simulink model "monopod_leg_force"  (R2013a)
settings: Solver=FixedStepDiscrete  StartTime=0.0  StopTime=inf  FixedStep=sample_time  RelTol=1e-3
InitFcn:
  | init_monopod_leg_force;
values from neighbouring files (symbols this model uses):
  sample_time = 1/update_freq    (= 0.001)    [init_monopod_leg_force.m]
undefined symbols (not defined in the file or in its folder): BOOM_MAX_ENCODER_TICKS, boom_mount_angle, BOOM_PITCH_CAL_VALUE_RAD, BOOM_PITCH_CAL_VALUE_TICKS, BOOM_PITCH_ENCODER_RAD_PER_TICK, BOOM_ROLL_CAL_VALUE_RAD, BOOM_ROLL_CAL_VALUE_TICKS, BOOM_ROLL_ENCODER_RAD_PER_TICK, BOOM_YAW_ENCODER_RAD_PER_TICK, control_start_time, DiscIntNeverNeededParam, fcut_acceleration, fcut_smooth, fcut_unwrap, fcut_velocity, HIP_ABS_ENCODER_RAD_PER_TICK, HIP_ABS_MAX_ENCODER_TICKS, hip_gravity_compensation, HIP_INC_ENCODER_RAD_PER_TICK, HIP_INC_MAX_ENCODER_TICKS, HIP_MOTOR_CONSTANT, HIP_MTR_GEAR_RATIO, HIP_MTR_MAX_TORQUE, i_limit_lateral, j_rotor_reflected, k_ff, k_sea, k_virtual, kd_lateral, kd_leg_angle, kd_sea_torque, ki_lateral, kp_lateral, kp_leg_angle, kp_sea_torque, l0_virtual, l_seg, lateral_torque_ramp_time, LEFT_HIP_CALIB_POS, LEFT_HIP_CALIB_VAL, LEFT_MOTOR_HIP_DIRECTION, LEG1_LEG_A_CALIB_VAL, LEG1_LEG_A_RAD_PER_CNT, LEG1_LEG_B_CALIB_VAL, LEG1_LEG_B_RAD_PER_CNT, LEG1_MOTOR_A_DIRECTION, LEG1_MOTOR_B_DIRECTION, LEG1_TRAN_A_CALIB_VAL, LEG1_TRAN_A_RAD_PER_CNT, LEG1_TRAN_B_CALIB_VAL, LEG1_TRAN_B_RAD_PER_CNT, LEG2_LEG_A_CALIB_VAL, LEG2_LEG_A_RAD_PER_CNT, LEG2_LEG_B_CALIB_VAL, LEG2_LEG_B_RAD_PER_CNT, LEG2_MOTOR_A_DIRECTION, LEG2_MOTOR_B_DIRECTION, LEG2_TRAN_A_CALIB_VAL, LEG2_TRAN_A_RAD_PER_CNT, LEG2_TRAN_B_CALIB_VAL ... (+18)
libraries: xpcethercatlib x160, simulink x13, dspswit3 x1
(part 3 of 3)

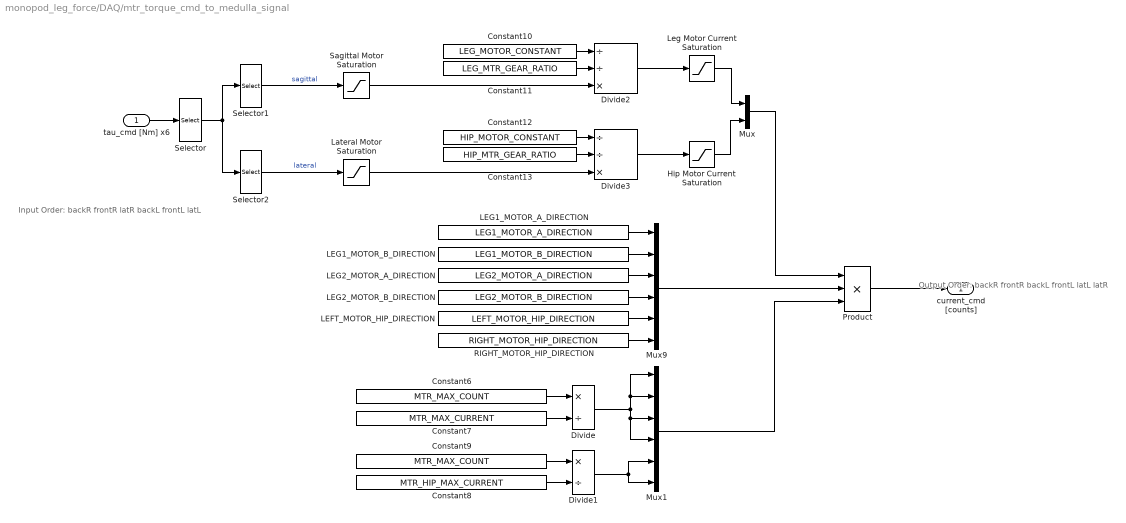
== system monopod_leg_force/DAQ/mtr_torque_cmd_to_medulla_signal ==
  note: Output Order:
      |
      | backR
      | frontR
      | backL
      | frontL
      | latL
      | latR
  note: Input Order:
      |
      | backR
      | frontR
      | latR
      | backL
      | frontL
      | latL
  tau_cmd [Nm] x6 : Inport
  Constant10 : Constant  Value=LEG_MOTOR_CONSTANT
  Constant11 : Constant  Value=LEG_MTR_GEAR_RATIO
  Constant12 : Constant  Value=HIP_MOTOR_CONSTANT
  Constant13 : Constant  Value=HIP_MTR_GEAR_RATIO
  Constant6 : Constant  Value=MTR_MAX_COUNT
  Constant7 : Constant  Value=MTR_MAX_CURRENT
  Constant8 : Constant  Value=MTR_HIP_MAX_CURRENT
  Constant9 : Constant  Value=MTR_MAX_COUNT
  Divide : Product  Inputs=*/
  Divide1 : Product  Inputs=*/
  Divide2 : Product  Inputs=//*
  Divide3 : Product  Inputs=//*
  Hip Motor Current Saturation : Saturate  UpperLimit=10  LowerLimit=-10
      settings: AttributesFormatString=Top: %<UpperLimit>\nBottom: %<LowerLimit>
  LEFT_MOTOR_HIP_DIRECTION : Constant  Value=LEFT_MOTOR_HIP_DIRECTION
  LEG1_MOTOR_A_DIRECTION : Constant  Value=LEG1_MOTOR_A_DIRECTION
  LEG1_MOTOR_B_DIRECTION : Constant  Value=LEG1_MOTOR_B_DIRECTION
  LEG2_MOTOR_A_DIRECTION : Constant  Value=LEG2_MOTOR_A_DIRECTION
  LEG2_MOTOR_B_DIRECTION : Constant  Value=LEG2_MOTOR_B_DIRECTION
  Lateral Motor Saturation : Saturate  UpperLimit=HIP_MTR_MAX_TORQUE  LowerLimit=-HIP_MTR_MAX_TORQUE
      settings: AttributesFormatString=Top: %<UpperLimit>\nBottom: %<LowerLimit>
  Leg Motor Current Saturation : Saturate  UpperLimit=30  LowerLimit=-30
      settings: AttributesFormatString=Top: %<UpperLimit>\nBottom: %<LowerLimit>
  Mux : Mux  Inputs=2
  Mux1 : Mux  Inputs=6
  Mux9 : Mux  Inputs=6
  Product : Product  Inputs=3  RndMeth=Zero
  RIGHT_MOTOR_HIP_DIRECTION : Constant  Value=RIGHT_MOTOR_HIP_DIRECTION
  Sagittal Motor Saturation : Saturate  UpperLimit=LEG_MTR_MAX_TORQUE  LowerLimit=-LEG_MTR_MAX_TORQUE
      settings: AttributesFormatString=Top: %<UpperLimit>\nBottom: %<LowerLimit>
  Selector : Selector  InputPortWidth=6  IndexOptions=Index vector (dialog)  Indices=[1 2 4 5 6 3]  OutputSizes=1
  Selector1 : Selector  InputPortWidth=6  IndexOptions=Index vector (dialog)  Indices=[1 2 3 4]  OutputSizes=1
  Selector2 : Selector  InputPortWidth=6  IndexOptions=Index vector (dialog)  Indices=[5 6]  OutputSizes=1
  current_cmd [counts] : Outport
  wires:
  Lateral Motor Saturation/1 -> Divide3/3
  Sagittal Motor Saturation/1 -> Divide2/3
  Hip Motor Current Saturation/1 -> Mux/2
  Leg Motor Current Saturation/1 -> Mux/1
  Mux/1 -> Product/1
  Divide2/1 -> Leg Motor Current Saturation/1
  Divide3/1 -> Hip Motor Current Saturation/1
  Constant12/1 -> Divide3/1
  Constant13/1 -> Divide3/2
  Constant10/1 -> Divide2/1
  Constant11/1 -> Divide2/2
  Selector2/1 -> Lateral Motor Saturation/1  "lateral"
  Selector1/1 -> Sagittal Motor Saturation/1  "sagittal"
  LEG1_MOTOR_A_DIRECTION/1 -> Mux9/1
  LEG1_MOTOR_B_DIRECTION/1 -> Mux9/2
  LEG2_MOTOR_A_DIRECTION/1 -> Mux9/3
  Mux9/1 -> Product/2
  LEG2_MOTOR_B_DIRECTION/1 -> Mux9/4
  LEFT_MOTOR_HIP_DIRECTION/1 -> Mux9/5
  RIGHT_MOTOR_HIP_DIRECTION/1 -> Mux9/6
  Product/1 -> current_cmd [counts]/1
  Constant6/1 -> Divide/1
  Constant7/1 -> Divide/2
  Divide/1 -> Mux1/4, Mux1/3, Mux1/2, Mux1/1
  Constant9/1 -> Divide1/1
  Constant8/1 -> Divide1/2
  Divide1/1 -> Mux1/6, Mux1/5
  Mux1/1 -> Product/3
  tau_cmd [Nm] x6/1 -> Selector/1
  Selector/1 -> Selector1/1, Selector2/1

== system monopod_leg_force/DAQ/remove_encoder_dropouts ==
  note: Predict Behavior of Signal
  note: predicted value:
      | phi' = phi_(n-1) + dphi
      | = phi_(n-1) + phi_(n-1)-phi_(n-2)
  measured : Inport
  Abs : Abs
  Clock : Clock
  Compare To Zero1 : simulink/Logic and Bit Operations/Compare To Zero  relop=>  OutDataTypeStr=boolean
  Constant : Constant  Value=sensor_start_time+2*sample_time
  Discrete Single Pole Lowpass Filter : DiscreteTransferFcn  Numerator=[(1-exp(-2*pi*fcut_smooth*sample_time)) 0]  Denominator=[1 -exp(-2*pi*fcut_smooth*sample_time)]  SampleTime=sample_time
  Gain2 : Gain  Gain=2
  Sum : Sum  Inputs=|+-
  Sum2 : Sum  Inputs=|+-
  Sum3 : Sum  Inputs=-+|
  Switch : Switch  Criteria=u2 ~= 0  Threshold=max_sensor_velocity*sample_time
      settings: AttributesFormatString=%<Criteria>
  Unit Delay phi_(n-1) : UnitDelay  SampleTime=-1
      settings: AttributesFormatString=initial condition = %<X0>
  Unit Delay phi_(n-2) : UnitDelay  SampleTime=-1
      settings: AttributesFormatString=initial condition = %<X0>
  check_error : Subsystem
  smoothed : Outport
  wires:
  Compare To Zero1/1 -> check_error/Enable
  Constant/1 -> Sum2/2
  Clock/1 -> Sum2/1
  Sum2/1 -> Compare To Zero1/1
  check_error/1(acceptable?) -> Switch/2
  Sum3/1 -> Abs/1  "error"
  Abs/1 -> check_error/1(error)
  Discrete Single Pole Lowpass Filter/1 -> Unit Delay phi_(n-1)/1
  Switch/1 -> smoothed/1, Discrete Single Pole Lowpass Filter/1
  Unit Delay phi_(n-2)/1 -> Sum/2
  measured/1 -> Switch/1, Sum3/1  "phi"
  Unit Delay phi_(n-1)/1 -> Unit Delay phi_(n-2)/1, Gain2/1
  Gain2/1 -> Sum/1
  Sum/1 -> Sum3/2, Switch/3  "phi'"

== system monopod_leg_force/DAQ/unwrap_encoders ==
  Encoder Readings : Inport
  Demux : Demux  Outputs=5
  Mux : Mux  Inputs=6
  Selector : Selector  InputPortWidth=15  IndexOptions=Index vector (dialog)  Indices=[9 10 11 12 14]  OutputSizes=1
  Selector1 : Selector  InputPortWidth=20  IndexOptions=Index vector (dialog)  Indices=[1 2 3 4 5 6 7 8 16 17 18 19 13 20 15]  OutputSizes=1
  unwrap_boom_yaw_encoder : Subsystem
  unwrap_lateral_absolute_encoders Left : Subsystem
  unwrap_lateral_absolute_encoders Right : Subsystem
  unwrap_lateral_incremental_encoders Left : Subsystem
  unwrap_lateral_incremental_encoders Right : Subsystem
  Adjusted Encoder Readings : Outport
  wires:
  Encoder Readings/1 -> Mux/1, Selector/1
  Selector/1 -> Demux/1
  Demux/2 -> unwrap_lateral_incremental_encoders Left/1(wrapped [ticks])
  Demux/4 -> unwrap_lateral_incremental_encoders Right/1(wrapped [ticks])
  Demux/5 -> unwrap_boom_yaw_encoder/1(wrapped [ticks])
  unwrap_lateral_incremental_encoders Left/1(continuous [ticks]) -> Mux/3
  unwrap_lateral_incremental_encoders Right/1(continuous [ticks]) -> Mux/5
  unwrap_boom_yaw_encoder/1(continuous [ticks]) -> Mux/6
  Selector1/1 -> Adjusted Encoder Readings/1
  Mux/1 -> Selector1/1
  Demux/1 -> unwrap_lateral_absolute_encoders Left/1(wrapped [ticks])
  Demux/3 -> unwrap_lateral_absolute_encoders Right/1(wrapped [ticks])
  unwrap_lateral_absolute_encoders Right/1(continuous [ticks]) -> Mux/4
  unwrap_lateral_absolute_encoders Left/1(continuous [ticks]) -> Mux/2

== system monopod_leg_force/Control/Actuator Control/SEA Controller ==
  phi_load [rad] x4 : Inport
  phi_gear [rad] x4 : Inport  Port=2
  tau_des sagittal [Nm] x4 : Inport  Port=3
  dphi_load [rad/s] x4 : Inport  Port=4
  dphi_gear [rad/s] x4 : Inport  Port=5
  Constant : Constant  Value=0
  Constant1 : Constant  Value=0
  Constant3 : Constant
  Product : Product  SampleTime=sample_time  RndMeth=Zero
  Product1 : Product  RndMeth=Zero
  Spring Stiffness : Gain  Gain=k_sea
  Spring Stiffness1 : Gain  Gain=k_sea
  Sum : Sum  Inputs=|++  SampleTime=sample_time
  Sum1 : Sum  Inputs=-+|
  Sum2 : Sum  Inputs=|+-
  Sum3 : Sum  Inputs=+++
  Sum5 : Sum  Inputs=|+-
  Sum6 : Sum  Inputs=-+|
  Sum7 : Sum  Inputs=|++
  Torque Limiter (outside) 1 : Saturate  UpperLimit=max_sagittal_torque  LowerLimit=-max_sagittal_torque
      settings: AttributesFormatString=Hi: %<UpperLimit>\nLo: %<LowerLimit>
  filtered_derivative : Subsystem
  j_motor : Gain  Description=xPCTag(1)=kd_sea_torque;  Gain=j_rotor_reflected
  k_ff : Gain  Gain=k_ff
  kd_gain : Gain  Description=xPCTag(1)=kd_sea_torque;  Gain=kd_sea_torque
  kp_gain : Constant  Description=xPCTag(1)=kp_sea_torque;  Value=kp_sea_torque  SampleTime=sample_time
  tau_cmd sagittal [Nm] x4 : Outport
  wires:
  Torque Limiter (outside) 1/1 -> tau_cmd sagittal [Nm] x4/1
  j_motor/1 -> k_ff/1
  filtered_derivative/1(dx/dt) -> j_motor/1
  Sum/1 -> Product1/2
  Constant3/1 -> Sum/2
  Sum7/1 -> Sum3/2
  kd_gain/1 -> Sum7/2
  Product/1 -> Sum7/1
  Sum5/1 -> Product/2
  Sum2/1 -> kd_gain/1
  dphi_gear [rad/s] x4/1 -> Sum6/2
  dphi_load [rad/s] x4/1 -> filtered_derivative/1(x), Sum6/1
  Spring Stiffness1/1 -> Sum2/2
  Sum6/1 -> Spring Stiffness1/1
  Constant1/1 -> Sum2/1
  Constant/1 -> Sum5/1
  phi_gear [rad] x4/1 -> Sum1/2
  phi_load [rad] x4/1 -> Sum1/1
  Sum3/1 -> Torque Limiter (outside) 1/1
  Product1/1 -> Sum3/1
  tau_des sagittal [Nm] x4/1 -> Product1/1
  Spring Stiffness/1 -> Sum5/2
  Sum1/1 -> Spring Stiffness/1
  kp_gain/1 -> Sum/1, Product/1
  k_ff/1 -> Sum3/3

== system monopod_leg_force/Control/Actuator Control/ramped_signal ==
  cmd : Inport
  Constant : Constant  Value=0
  Demux : Demux
  Mux1 : Mux
  Mux6 : Mux  Inputs=2
  Product : Product  RndMeth=Zero
  Product1 : Product  RndMeth=Zero
  Ramp : simulink/Sources/Ramp  slope=1/sagittal_torque_ramp_time  start=sagittal_starting_time  X0=0
      settings: AttributesFormatString=Start: %<start>\nSlope: %<slope>
  Ramp1 : simulink/Sources/Ramp  slope=1/lateral_torque_ramp_time  start=control_start_time  X0=0
      settings: AttributesFormatString=Start: %<start>\nSlope: %<slope>
  Saturation : Saturate  UpperLimit=1  LowerLimit=0
      settings: AttributesFormatString=Hi: %<UpperLimit>\nLo: %<LowerLimit>
  Saturation1 : Saturate  UpperLimit=1  LowerLimit=0
      settings: AttributesFormatString=Hi: %<UpperLimit>\nLo: %<LowerLimit>
  Selector10 : Selector  InputPortWidth=6  IndexOptions=Index vector (dialog)  Indices=[1 2 4 5]  OutputSizes=1
  Selector34 : Selector  InputPortWidth=6  IndexOptions=Index vector (dialog)  Indices=[1 2 5 3 4 6]  OutputSizes=1
  Selector9 : Selector  InputPortWidth=6  IndexOptions=Index vector (dialog)  Indices=[3 6]  OutputSizes=1
  Terminator : Terminator
  Terminator1 : Terminator
  ramped_cmd : Outport
  wires:
  Demux/3 -> Terminator1/1
  Demux/4 -> Terminator/1
  Constant/1 -> Mux1/4, Mux1/3
  Mux1/1 -> Product/1
  Demux/2 -> Mux1/2
  Demux/1 -> Mux1/1
  Mux6/1 -> Selector34/1
  Selector10/1 -> Demux/1
  Selector34/1 -> ramped_cmd/1
  Product1/1 -> Mux6/2
  cmd/1 -> Selector9/1, Selector10/1
  Product/1 -> Mux6/1
  Ramp/1 -> Saturation/1
  Saturation/1 -> Product/2
  Ramp1/1 -> Saturation1/1
  Saturation1/1 -> Product1/2
  Selector9/1 -> Product1/1

== system monopod_leg_force/Control/Behavior Control/Lateral PID Control ==
  q_cmu : Inport
  dq_cmu : Inport  Port=2
  Gain : Gain  Gain=-1
  Lateral Hip PID : Subsystem
  Motor Saturation : Saturate  UpperLimit=max_torque_lateral  LowerLimit=-max_torque_lateral
      settings: AttributesFormatString=Top: %<UpperLimit>\nBottom: %<LowerLimit>
  Mux : Mux  Inputs=2
  Sum1 : Sum  Inputs=|+-
  Sum2 : Sum  Inputs=|+-
  Sum4 : Sum  Inputs=++|
  desired_velocity : Constant  Value=0
  feedforward_torque (gravity compensation) : Constant  Value=hip_gravity_compensation
  select_dqLateral : Selector  InputPortWidth=13  IndexOptions=Index vector (dialog)  Indices=[9 10]  OutputSizes=1
  select_qLateral : Selector  InputPortWidth=13  IndexOptions=Index vector (dialog)  Indices=[9 10]  OutputSizes=1
  spherical_correction_angle : Subsystem
  tau_lateral : Outport
  wires:
  spherical_correction_angle/1(lateral_correction [rad]) -> Mux/1, Gain/1
  Lateral Hip PID/1(out) -> Sum4/2
  Sum2/1 -> Lateral Hip PID/1(position_error)
  q_cmu/1 -> spherical_correction_angle/1(q_cmu), select_qLateral/1
  select_dqLateral/1 -> Sum1/2
  dq_cmu/1 -> select_dqLateral/1
  Sum4/1 -> Motor Saturation/1
  desired_velocity/1 -> Sum1/1
  Sum1/1 -> Lateral Hip PID/2(velocity_error)
  feedforward_torque (gravity compensation)/1 -> Sum4/1
  Gain/1 -> Mux/2
  Mux/1 -> Sum2/1
  select_qLateral/1 -> Sum2/2  "qLateral"
  Motor Saturation/1 -> tau_lateral/1

== system monopod_leg_force/Control/Behavior Control/Leg Calculator ==
  Front [rad rad/s] : Inport
  Back [rad rad/s] : Inport  Port=2
  Demux1 : Demux  Outputs=2
  Gain1 : Gain  Gain=2*l_seg
  Gain2 : Gain  Gain=l_seg
  Gain3 : Gain  Gain=-1
  Gain4 : Gain  Gain=0.5
  Gain5 : Gain  Gain=0.5
  Gain6 : Gain  Gain=2
  Mux1 : Mux  Inputs=2
  Product : Product  RndMeth=Zero
  Sum4 : Sum  Inputs=+|+
  Sum5 : Sum  Inputs=+|-
  Trigonometric Function : Trigonometry  Operator=cos
  Trigonometric Function1 : Trigonometry
  "Leg Length [m m/s] " : Outport
  Leg Angle [rad rad/s] : Outport  Port=2
  Leg Splay [rad rad/s] : Outport  Port=3
  w [m] : Outport  Port=4
  wires:
  Gain6/1 -> w [m]/1
  Gain4/1 -> Trigonometric Function1/1, Trigonometric Function/1
  Trigonometric Function/1 -> Gain1/1
  Gain1/1 -> Mux1/1
  Trigonometric Function1/1 -> Gain2/1
  Product/1 -> Mux1/2
  Front [rad rad/s]/1 -> Sum5/2, Sum4/2
  Back [rad rad/s]/1 -> Sum4/1, Sum5/1
  Demux1/2 -> Gain3/1
  Gain3/1 -> Product/2
  Demux1/1 -> Gain4/1
  Gain2/1 -> Product/1, Gain6/1
  Sum5/1 -> Leg Splay [rad rad/s]/1, Demux1/1
  Mux1/1 -> "Leg Length [m m/s] "/1
  Sum4/1 -> Gain5/1
  Gain5/1 -> Leg Angle [rad rad/s]/1

== system monopod_leg_force/Control/Behavior Control/R Leg Angle PD ==
  Desired Angle : Inport
  Desired Velocity : Inport  Port=2
  Leg Angle [rad rad/s] : Inport  Port=3
  Demux1 : Demux  Outputs=2
  Gain6 : Gain  Gain=kp_leg_angle
  Gain7 : Gain  Gain=kd_leg_angle
  Sum7 : Sum  Inputs=|+-
  Sum8 : Sum  Inputs=|+-
  Sum9 : Sum  Inputs=|++
  Commanded Leg Torque [Nm] : Outport
  wires:
  Sum7/1 -> Gain6/1
  Demux1/1 -> Sum7/2
  Sum9/1 -> Commanded Leg Torque [Nm]/1
  Desired Velocity/1 -> Sum8/1
  Sum8/1 -> Gain7/1
  Desired Angle/1 -> Sum7/1
  Demux1/2 -> Sum8/2
  Leg Angle [rad rad/s]/1 -> Demux1/1
  Gain6/1 -> Sum9/1
  Gain7/1 -> Sum9/2

== system monopod_leg_force/Control/Behavior Control/Torque Distribution ==
  Leg Torque [Nm] : Inport
  Leg Force [N] : Inport  Port=2
  Leg Splay [rad] : Inport  Port=3
  Gain : Gain  Gain=0.5
  Gain1 : Gain  Gain=0.5
  Gain2 : Gain  Gain=2*l_seg
  Gain3 : Gain  Gain=0.5
  Product : Product  RndMeth=Zero
  Sum : Sum  Inputs=|++
  Sum1 : Sum  Inputs=+-|
  Trigonometric Function1 : Trigonometry
  Back Torque [Nm] : Outport
  Front Torque [Nm] : Outport  Port=2
  wires:
  Sum1/1 -> Back Torque [Nm]/1
  Leg Torque [Nm]/1 -> Gain/1
  Sum/1 -> Front Torque [Nm]/1
  Gain/1 -> Sum/1, Sum1/1
  Gain3/1 -> Trigonometric Function1/1
  Leg Splay [rad]/1 -> Gain3/1
  Trigonometric Function1/1 -> Gain2/1
  Gain2/1 -> Product/2  "w [m]"
  Gain1/1 -> Sum1/2, Sum/2
  Leg Force [N]/1 -> Product/1
  Product/1 -> Gain1/1

== system monopod_leg_force/DAQ/calibrate_and_convert_to_rad/calibrate_abs_encoder ==
  encoder_ticks : Inport
  cal_pt_ticks : Inport  Port=2
  cal_pt_rad : Inport  Port=3
  ticks_to_rad_const : Inport  Port=4
  Product : Product  RndMeth=Zero
  Sum : Sum  Inputs=|+-
  Sum1 : Sum  Inputs=|++
  angle [rad] : Outport
  wires:
  cal_pt_rad/1 -> Sum1/2  "calibration_point_radians"
  Sum1/1 -> angle [rad]/1  "calibrated_angle"
  cal_pt_ticks/1 -> Sum/2  "calibration_point_ticks"
  ticks_to_rad_const/1 -> Product/2  "ticks_to_rad_const"
  Product/1 -> Sum1/1  "rad_diff"
  encoder_ticks/1 -> Sum/1  "encoder_ticks"
  Sum/1 -> Product/1  "tick_diff"

== system monopod_leg_force/DAQ/calibrate_and_convert_to_rad/calibration_pt_radians ==
  Constant{1,3,5,7} (4 alike) : Constant  Value=LEG_A_CALIB_LOC
  Constant10 : Constant  Value=LEFT_HIP_CALIB_POS
  Constant11 : Constant  Value=BOOM_ROLL_CAL_VALUE_RAD
  Constant12 : Constant  Value=BOOM_PITCH_CAL_VALUE_RAD
  Constant{2,4,6,8} (4 alike) : Constant  Value=LEG_B_CALIB_LOC
  Constant9 : Constant  Value=RIGHT_HIP_CALIB_POS
  Mux3 : Mux  Inputs=12
  calibration_pt [rad] : Outport
  wires:
  Constant7/1 -> Mux3/5
  Constant10/1 -> Mux3/9
  Constant1/1 -> Mux3/2
  Constant5/1 -> Mux3/6
  Constant2/1 -> Mux3/3
  Constant9/1 -> Mux3/10
  Constant12/1 -> Mux3/12
  Constant6/1 -> Mux3/7
  Constant11/1 -> Mux3/11
  Mux3/1 -> calibration_pt [rad]/1
  Constant3/1 -> Mux3/1
  Constant8/1 -> Mux3/8
  Constant4/1 -> Mux3/4

== system monopod_leg_force/DAQ/calibrate_and_convert_to_rad/calibration_pt_ticks ==
  Constant1 : Constant  Value=LEG2_TRAN_A_CALIB_VAL
  Constant10 : Constant  Value=LEFT_HIP_CALIB_VAL
  Constant11 : Constant  Value=BOOM_ROLL_CAL_VALUE_TICKS
  Constant12 : Constant  Value=BOOM_PITCH_CAL_VALUE_TICKS
  Constant2 : Constant  Value=LEG2_LEG_B_CALIB_VAL
  Constant3 : Constant  Value=LEG2_LEG_A_CALIB_VAL
  Constant4 : Constant  Value=LEG2_TRAN_B_CALIB_VAL
  Constant5 : Constant  Value=LEG1_TRAN_A_CALIB_VAL
  Constant6 : Constant  Value=LEG1_LEG_B_CALIB_VAL
  Constant7 : Constant  Value=LEG1_LEG_A_CALIB_VAL
  Constant8 : Constant  Value=LEG1_TRAN_B_CALIB_VAL
  Constant9 : Constant  Value=RIGHT_HIP_CALIB_VAL
  Mux3 : Mux  Inputs=12
  calibration_pt [ticks] : Outport
  wires:
  Constant8/1 -> Mux3/4
  Constant4/1 -> Mux3/8
  Constant7/1 -> Mux3/1
  Mux3/1 -> calibration_pt [ticks]/1
  Constant11/1 -> Mux3/11
  Constant2/1 -> Mux3/7
  Constant12/1 -> Mux3/12
  Constant9/1 -> Mux3/10
  Constant6/1 -> Mux3/3
  Constant1/1 -> Mux3/6
  Constant5/1 -> Mux3/2
  Constant10/1 -> Mux3/9
  Constant3/1 -> Mux3/5

== system monopod_leg_force/DAQ/calibrate_and_convert_to_rad/ticks_to_radians_constants ==
  Constant1 : Constant  Value=LEG2_TRAN_A_RAD_PER_CNT
  Constant10 : Constant  Value=-HIP_ABS_ENCODER_RAD_PER_TICK
  Constant11 : Constant  Value=BOOM_ROLL_ENCODER_RAD_PER_TICK
  Constant12 : Constant  Value=BOOM_PITCH_ENCODER_RAD_PER_TICK
  Constant2 : Constant  Value=LEG2_LEG_B_RAD_PER_CNT
  Constant3 : Constant  Value=LEG2_LEG_A_RAD_PER_CNT
  Constant4 : Constant  Value=LEG2_TRAN_B_RAD_PER_CNT
  Constant5 : Constant  Value=LEG1_TRAN_A_RAD_PER_CNT
  Constant6 : Constant  Value=LEG1_LEG_B_RAD_PER_CNT
  Constant7 : Constant  Value=LEG1_LEG_A_RAD_PER_CNT
  Constant8 : Constant  Value=LEG1_TRAN_B_RAD_PER_CNT
  Constant9 : Constant  Value=HIP_ABS_ENCODER_RAD_PER_TICK
  Mux3 : Mux  Inputs=12
  ticks_to_rad_constants : Outport
  wires:
  Constant8/1 -> Mux3/4
  Constant4/1 -> Mux3/8
  Constant7/1 -> Mux3/1
  Mux3/1 -> ticks_to_rad_constants/1
  Constant11/1 -> Mux3/11
  Constant2/1 -> Mux3/7
  Constant12/1 -> Mux3/12
  Constant10/1 -> Mux3/10
  Constant6/1 -> Mux3/3
  Constant1/1 -> Mux3/6
  Constant5/1 -> Mux3/2
  Constant9/1 -> Mux3/9
  Constant3/1 -> Mux3/5

== system monopod_leg_force/DAQ/hold_initial_lateral_angles/Initial Lateral Hip Angles [rad] ==
  In : Inport
  Enable : EnablePort  StatesWhenEnabling=reset
  Out : Outport
  wires:
  In/1 -> Out/1

== system monopod_leg_force/DAQ/remove_encoder_dropouts/check_error ==
  error : Inport
  Enable : EnablePort
  Compare To Constant : simulink/Logic and Bit Operations/Compare To Constant  relop=<=  const=max_encoder_velocity*sample_time  OutDataTypeStr=boolean
  acceptable? : Outport  InitialOutput=1
  wires:
  Compare To Constant/1 -> acceptable?/1
  error/1 -> Compare To Constant/1

== system monopod_leg_force/DAQ/unwrap_encoders/unwrap_boom_yaw_encoder ==
  note: predicted angle:
      | phi' = phi_(n-1) + dphi
      | = phi_(n-1) + phi_(n-1)-phi_(n-2)
  note: Transform Wrapped Angle into Continuous Angle
  note: Recommended if-then structure for assigning
      | constants. The criterion '~=0' is realized as cpu register
      | shift when compiling.  The resulting code is fast.
  wrapped [ticks] : Inport
  1/BOOM_MAX_ENCODER_TICKS : Gain  Gain=1/BOOM_MAX_ENCODER_TICKS
  Abs : Abs
  BOOM_MAX_ENCODER_TICKS : Gain  Gain=BOOM_MAX_ENCODER_TICKS
  Compare To Zero : simulink/Logic and Bit Operations/Compare To Zero  relop=>  OutDataTypeStr=uint8
  Discrete Single Pole Lowpass Filter : DiscreteTransferFcn  Numerator=[(1-exp(-2*pi*fcut_unwrap*sample_time)) 0]  Denominator=[1 -exp(-2*pi*fcut_unwrap*sample_time)]  SampleTime=sample_time
  Gain2 : Gain  Gain=2
  Product : Product  RndMeth=Zero
  Rounding Function : Rounding
  Sum : Sum  Inputs=|+-
  Sum1 : Sum  Inputs=|++
  Sum2 : Sum  Inputs=|++
  Sum3 : Sum  Inputs=-+|
  Switch : Switch  Criteria=u2 ~= 0
      settings: AttributesFormatString=%<Criteria>
  Unit Delay phi_(n-1) : UnitDelay  SampleTime=-1
      settings: AttributesFormatString=initial condition = %<X0>
  Unit Delay phi_(n-2) : UnitDelay  SampleTime=-1
      settings: AttributesFormatString=initial condition = %<X0>
  const : Constant  Value=0.5
  no : Constant  Value=-1
  yes : Constant
  continuous [ticks] : Outport
  wires:
  Sum3/1 -> Compare To Zero/1, Abs/1  "phi'-phi"
  Sum/1 -> Sum3/2
  Gain2/1 -> Sum/1
  Unit Delay phi_(n-1)/1 -> Gain2/1, Unit Delay phi_(n-2)/1
  BOOM_MAX_ENCODER_TICKS/1 -> Product/1
  Sum1/1 -> Discrete Single Pole Lowpass Filter/1, continuous [ticks]/1
  Sum2/1 -> Rounding Function/1
  const/1 -> Sum2/2
  1/BOOM_MAX_ENCODER_TICKS/1 -> Sum2/1
  Abs/1 -> 1/BOOM_MAX_ENCODER_TICKS/1
  Product/1 -> Sum1/2
  wrapped [ticks]/1 -> Sum3/1, Sum1/1
  Rounding Function/1 -> BOOM_MAX_ENCODER_TICKS/1
  Switch/1 -> Product/2
  no/1 -> Switch/3
  yes/1 -> Switch/1
  Unit Delay phi_(n-2)/1 -> Sum/2
  Compare To Zero/1 -> Switch/2
  Discrete Single Pole Lowpass Filter/1 -> Unit Delay phi_(n-1)/1

== system monopod_leg_force/DAQ/unwrap_encoders/unwrap_lateral_absolute_encoders Left ==
  note: Recommended if-then structure for assigning
      | constants. The criterion '~=0' is realized as cpu register
      | shift when compiling.  The resulting code is fast.
  note: Transform Wrapped Angle into Continuous Angle
  note: predicted angle:
      | phi' = phi_(n-1) + dphi
      | = phi_(n-1) + phi_(n-1)-phi_(n-2)
  wrapped [ticks] : Inport
  1/HIP_ABS_MAX_ENCODER_TICKS : Gain  Gain=1/HIP_ABS_MAX_ENCODER_TICKS
  Abs : Abs
  Compare To Zero : simulink/Logic and Bit Operations/Compare To Zero  relop=>  OutDataTypeStr=uint8
  Discrete Single Pole Lowpass Filter : DiscreteTransferFcn  Numerator=[(1-exp(-2*pi*fcut_unwrap*sample_time)) 0]  Denominator=[1 -exp(-2*pi*fcut_unwrap*sample_time)]  SampleTime=sample_time
  Gain2 : Gain  Gain=2
  HIP_ABS_MAX_ENCODER_TICKS : Gain  Gain=HIP_ABS_MAX_ENCODER_TICKS
  Product : Product  RndMeth=Zero
  Rounding Function : Rounding
  Sum : Sum  Inputs=|+-
  Sum1 : Sum  Inputs=|++
  Sum2 : Sum  Inputs=|++
  Sum3 : Sum  Inputs=-+|
  Switch : Switch  Criteria=u2 ~= 0
      settings: AttributesFormatString=%<Criteria>
  Unit Delay phi_(n-1) : UnitDelay  SampleTime=-1
      settings: AttributesFormatString=initial condition = %<X0>
  Unit Delay phi_(n-2) : UnitDelay  SampleTime=-1
      settings: AttributesFormatString=initial condition = %<X0>
  const : Constant  Value=0.5
  no : Constant  Value=-1
  yes : Constant
  continuous [ticks] : Outport
  wires:
  Discrete Single Pole Lowpass Filter/1 -> Unit Delay phi_(n-1)/1
  Compare To Zero/1 -> Switch/2
  Unit Delay phi_(n-2)/1 -> Sum/2
  yes/1 -> Switch/1
  no/1 -> Switch/3
  Switch/1 -> Product/2
  Rounding Function/1 -> HIP_ABS_MAX_ENCODER_TICKS/1
  wrapped [ticks]/1 -> Sum1/1, Sum3/1
  Product/1 -> Sum1/2
  Abs/1 -> 1/HIP_ABS_MAX_ENCODER_TICKS/1
  1/HIP_ABS_MAX_ENCODER_TICKS/1 -> Sum2/1
  const/1 -> Sum2/2
  Sum2/1 -> Rounding Function/1
  Sum1/1 -> Discrete Single Pole Lowpass Filter/1, continuous [ticks]/1
  HIP_ABS_MAX_ENCODER_TICKS/1 -> Product/1
  Unit Delay phi_(n-1)/1 -> Unit Delay phi_(n-2)/1, Gain2/1
  Gain2/1 -> Sum/1
  Sum/1 -> Sum3/2
  Sum3/1 -> Abs/1, Compare To Zero/1  "phi'-phi"

== system monopod_leg_force/DAQ/unwrap_encoders/unwrap_lateral_absolute_encoders Right ==
  note: predicted angle:
      | phi' = phi_(n-1) + dphi
      | = phi_(n-1) + phi_(n-1)-phi_(n-2)
  note: Transform Wrapped Angle into Continuous Angle
  note: Recommended if-then structure for assigning
      | constants. The criterion '~=0' is realized as cpu register
      | shift when compiling.  The resulting code is fast.
  wrapped [ticks] : Inport
  1/HIP_ABS_MAX_ENCODER_TICKS : Gain  Gain=1/HIP_ABS_MAX_ENCODER_TICKS
  Abs : Abs
  Compare To Zero : simulink/Logic and Bit Operations/Compare To Zero  relop=>  OutDataTypeStr=uint8
  Discrete Single Pole Lowpass Filter : DiscreteTransferFcn  Numerator=[(1-exp(-2*pi*fcut_unwrap*sample_time)) 0]  Denominator=[1 -exp(-2*pi*fcut_unwrap*sample_time)]  SampleTime=sample_time
  Gain2 : Gain  Gain=2
  HIP_ABS_MAX_ENCODER_TICKS : Gain  Gain=HIP_ABS_MAX_ENCODER_TICKS
  Product : Product  RndMeth=Zero
  Rounding Function : Rounding
  Sum : Sum  Inputs=|+-
  Sum1 : Sum  Inputs=|++
  Sum2 : Sum  Inputs=|++
  Sum3 : Sum  Inputs=-+|
  Switch : Switch  Criteria=u2 ~= 0
      settings: AttributesFormatString=%<Criteria>
  Unit Delay phi_(n-1) : UnitDelay  SampleTime=-1
      settings: AttributesFormatString=initial condition = %<X0>
  Unit Delay phi_(n-2) : UnitDelay  SampleTime=-1
      settings: AttributesFormatString=initial condition = %<X0>
  const : Constant  Value=0.5
  no : Constant  Value=-1
  yes : Constant
  continuous [ticks] : Outport
  wires:
  Sum3/1 -> Compare To Zero/1, Abs/1  "phi'-phi"
  Sum/1 -> Sum3/2
  Gain2/1 -> Sum/1
  Unit Delay phi_(n-1)/1 -> Gain2/1, Unit Delay phi_(n-2)/1
  HIP_ABS_MAX_ENCODER_TICKS/1 -> Product/1
  Sum1/1 -> continuous [ticks]/1, Discrete Single Pole Lowpass Filter/1
  Sum2/1 -> Rounding Function/1
  const/1 -> Sum2/2
  1/HIP_ABS_MAX_ENCODER_TICKS/1 -> Sum2/1
  Abs/1 -> 1/HIP_ABS_MAX_ENCODER_TICKS/1
  Product/1 -> Sum1/2
  wrapped [ticks]/1 -> Sum3/1, Sum1/1
  Rounding Function/1 -> HIP_ABS_MAX_ENCODER_TICKS/1
  Switch/1 -> Product/2
  no/1 -> Switch/3
  yes/1 -> Switch/1
  Unit Delay phi_(n-2)/1 -> Sum/2
  Compare To Zero/1 -> Switch/2
  Discrete Single Pole Lowpass Filter/1 -> Unit Delay phi_(n-1)/1

== system monopod_leg_force/DAQ/unwrap_encoders/unwrap_lateral_incremental_encoders Left ==
  note: predicted angle:
      | phi' = phi_(n-1) + dphi
      | = phi_(n-1) + phi_(n-1)-phi_(n-2)
  note: Transform Wrapped Angle into Continuous Angle
  note: Recommended if-then structure for assigning
      | constants. The criterion '~=0' is realized as cpu register
      | shift when compiling.  The resulting code is fast.
  wrapped [ticks] : Inport
  1/HIP_INC_MAX_ENCODER_TICKS : Gain  Gain=1/HIP_INC_MAX_ENCODER_TICKS
  Abs : Abs
  Compare To Zero : simulink/Logic and Bit Operations/Compare To Zero  relop=>  OutDataTypeStr=uint8
  Discrete Single Pole Lowpass Filter : DiscreteTransferFcn  Numerator=[(1-exp(-2*pi*fcut_unwrap*sample_time)) 0]  Denominator=[1 -exp(-2*pi*fcut_unwrap*sample_time)]  SampleTime=sample_time
  Gain2 : Gain  Gain=2
  HIP_INC_MAX_ENCODER_TICKS : Gain  Gain=HIP_INC_MAX_ENCODER_TICKS
  Product : Product  RndMeth=Zero
  Rounding Function : Rounding
  Sum : Sum  Inputs=|+-
  Sum1 : Sum  Inputs=|++
  Sum2 : Sum  Inputs=|++
  Sum3 : Sum  Inputs=-+|
  Switch : Switch  Criteria=u2 ~= 0
      settings: AttributesFormatString=%<Criteria>
  Unit Delay phi_(n-1) : UnitDelay  SampleTime=-1
      settings: AttributesFormatString=initial condition = %<X0>
  Unit Delay phi_(n-2) : UnitDelay  SampleTime=-1
      settings: AttributesFormatString=initial condition = %<X0>
  const : Constant  Value=0.5
  no : Constant  Value=-1
  yes : Constant
  continuous [ticks] : Outport
  wires:
  Sum3/1 -> Compare To Zero/1, Abs/1  "phi'-phi"
  Sum/1 -> Sum3/2
  Gain2/1 -> Sum/1
  Unit Delay phi_(n-1)/1 -> Gain2/1, Unit Delay phi_(n-2)/1
  HIP_INC_MAX_ENCODER_TICKS/1 -> Product/1
  Sum1/1 -> continuous [ticks]/1, Discrete Single Pole Lowpass Filter/1
  Sum2/1 -> Rounding Function/1
  const/1 -> Sum2/2
  1/HIP_INC_MAX_ENCODER_TICKS/1 -> Sum2/1
  Abs/1 -> 1/HIP_INC_MAX_ENCODER_TICKS/1
  Product/1 -> Sum1/2
  wrapped [ticks]/1 -> Sum3/1, Sum1/1
  Rounding Function/1 -> HIP_INC_MAX_ENCODER_TICKS/1
  Switch/1 -> Product/2
  no/1 -> Switch/3
  yes/1 -> Switch/1
  Unit Delay phi_(n-2)/1 -> Sum/2
  Compare To Zero/1 -> Switch/2
  Discrete Single Pole Lowpass Filter/1 -> Unit Delay phi_(n-1)/1

== system monopod_leg_force/DAQ/unwrap_encoders/unwrap_lateral_incremental_encoders Right ==
  note: Recommended if-then structure for assigning
      | constants. The criterion '~=0' is realized as cpu register
      | shift when compiling.  The resulting code is fast.
  note: Transform Wrapped Angle into Continuous Angle
  note: predicted angle:
      | phi' = phi_(n-1) + dphi
      | = phi_(n-1) + phi_(n-1)-phi_(n-2)
  wrapped [ticks] : Inport
  1/HIP_INC_MAX_ENCODER_TICKS : Gain  Gain=1/HIP_INC_MAX_ENCODER_TICKS
  Abs : Abs
  Compare To Zero : simulink/Logic and Bit Operations/Compare To Zero  relop=>  OutDataTypeStr=uint8
  Discrete Single Pole Lowpass Filter : DiscreteTransferFcn  Numerator=[(1-exp(-2*pi*fcut_unwrap*sample_time)) 0]  Denominator=[1 -exp(-2*pi*fcut_unwrap*sample_time)]  SampleTime=sample_time
  Gain2 : Gain  Gain=2
  HIP_INC_MAX_ENCODER_TICKS : Gain  Gain=HIP_INC_MAX_ENCODER_TICKS
  Product : Product  RndMeth=Zero
  Rounding Function : Rounding
  Sum : Sum  Inputs=|+-
  Sum1 : Sum  Inputs=|++
  Sum2 : Sum  Inputs=|++
  Sum3 : Sum  Inputs=-+|
  Switch : Switch  Criteria=u2 ~= 0
      settings: AttributesFormatString=%<Criteria>
  Unit Delay phi_(n-1) : UnitDelay  SampleTime=-1
      settings: AttributesFormatString=initial condition = %<X0>
  Unit Delay phi_(n-2) : UnitDelay  SampleTime=-1
      settings: AttributesFormatString=initial condition = %<X0>
  const : Constant  Value=0.5
  no : Constant  Value=-1
  yes : Constant
  continuous [ticks] : Outport
  wires:
  Discrete Single Pole Lowpass Filter/1 -> Unit Delay phi_(n-1)/1
  Compare To Zero/1 -> Switch/2
  Unit Delay phi_(n-2)/1 -> Sum/2
  yes/1 -> Switch/1
  no/1 -> Switch/3
  Switch/1 -> Product/2
  Rounding Function/1 -> HIP_INC_MAX_ENCODER_TICKS/1
  wrapped [ticks]/1 -> Sum1/1, Sum3/1
  Product/1 -> Sum1/2
  Abs/1 -> 1/HIP_INC_MAX_ENCODER_TICKS/1
  1/HIP_INC_MAX_ENCODER_TICKS/1 -> Sum2/1
  const/1 -> Sum2/2
  Sum2/1 -> Rounding Function/1
  Sum1/1 -> Discrete Single Pole Lowpass Filter/1, continuous [ticks]/1
  HIP_INC_MAX_ENCODER_TICKS/1 -> Product/1
  Unit Delay phi_(n-1)/1 -> Unit Delay phi_(n-2)/1, Gain2/1
  Gain2/1 -> Sum/1
  Sum/1 -> Sum3/2
  Sum3/1 -> Abs/1, Compare To Zero/1  "phi'-phi"

== system monopod_leg_force/Control/Actuator Control/SEA Controller/filtered_derivative ==
  x : Inport
  Gain1 : Gain  Gain=1/sample_time
  difference : simulink/Discrete/Difference  ICPrevInput=0.0  InputProcessing=Inherited  OutMin=[]  OutMax=[]  OutDataType=fixdt(1, 16)  OutScaling=2^-10  DoSatur=off
  single_pole_filter : DiscreteTransferFcn  Numerator=[(1-exp(-2*pi*fcut_acceleration*sample_time)) 0]  Denominator=[1 -exp(-2*pi*fcut_acceleration*sample_time)]  SampleTime=sample_time
  dx/dt : Outport
  wires:
  single_pole_filter/1 -> dx/dt/1
  x/1 -> Gain1/1
  difference/1 -> single_pole_filter/1
  Gain1/1 -> difference/1

== system monopod_leg_force/Control/Behavior Control/Lateral PID Control/Lateral Hip PID ==
  position_error : Inport
  velocity_error : Inport  Port=2
  Discrete-Time Integrator : DiscreteIntegrator  IntegratorMethod=Integration: Trapezoidal  SampleTime=sample_time  LimitOutput=on  UpperSaturationLimit=i_limit_lateral  LowerSaturationLimit=-i_limit_lateral  ICPrevOutput=DiscIntNeverNeededParam  ICPrevScaledInput=DiscIntNeverNeededParam
  Proportional Gain : Gain  Description=xPCTag(1)=kp_lateral;  Gain=kp_lateral
  Proportional Gain1 : Gain  Description=xPCTag(1)=kd_lateral;  Gain=kd_lateral
  Proportional Gain2 : Gain  Description=xPCTag(1)=ki_lateral;  Gain=ki_lateral
  Sum : Sum  Inputs=+++
  out : Outport
  wires:
  velocity_error/1 -> Proportional Gain1/1
  Discrete-Time Integrator/1 -> Sum/3
  Proportional Gain2/1 -> Discrete-Time Integrator/1
  Proportional Gain/1 -> Sum/2
  position_error/1 -> Proportional Gain2/1, Proportional Gain/1
  Sum/1 -> out/1
  Proportional Gain1/1 -> Sum/1

== system monopod_leg_force/Control/Behavior Control/Lateral PID Control/spherical_correction_angle ==
  q_cmu : Inport
  Selector : Selector  InputPortWidth=13  IndexOptions=Index vector (dialog)  Indices=[11]  OutputSizes=1
  Sum1 : Sum  Inputs=|+-
  Terminator2 : Terminator
  boom_mount_angle : Constant  Value=boom_mount_angle
  lateral_correction : Gain  Gain=180/pi
  lateral_correction [rad] : Outport
  wires:
  Sum1/1 -> lateral_correction/1, lateral_correction [rad]/1
  Selector/1 -> Sum1/1  "qBoomRoll"
  q_cmu/1 -> Selector/1
  boom_mount_angle/1 -> Sum1/2
  lateral_correction/1 -> Terminator2/1
